simulink model "tanques"  (Simulink 4.00)
settings: Solver=ode45  StartTime=0.0  StopTime=300  MaxStep=0.01  RelTol=1e-3
settings Model: LastModifiedBy=Gui

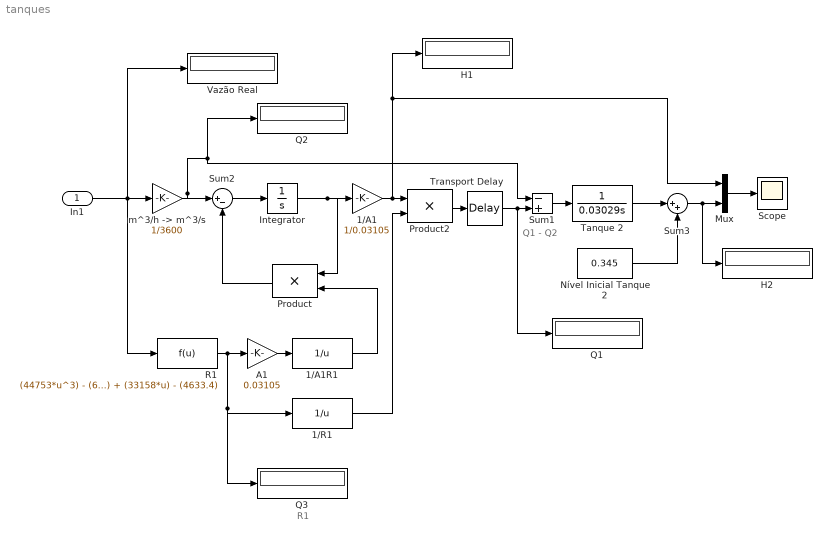
== system tanques ==
  note: Q1 - Q2
  note: R1
  In1 : Inport  Port=1  LatchInput=off
  1/A1 : Gain  Gain=1/0.03105  Multiplication=Element-wise(K.*u)  SaturateOnIntegerOverflow=on
  1/A1R1 : Fcn  Expr=1/u
  1/R1 : Fcn  Expr=1/u
  A1 : Gain  Gain=0.03105  Multiplication=Element-wise(K.*u)  SaturateOnIntegerOverflow=on
  H1 : Display
      settings: Format=short
  H2 : Display
      settings: Format=short
  Integrator : Integrator  ExternalReset=none  InitialConditionSource=internal  InitialCondition=0  LimitOutput=off  UpperSaturationLimit=inf  LowerSaturationLimit=-inf  ShowSaturationPort=off  ShowStatePort=off  AbsoluteTolerance=auto
  Mux : Mux  Inputs=2
  Nível Inicial Tanque 2 : Constant  Value=0.345
  Product : Product  Orientation=left  Inputs=2  Multiplication=Element-wise(.*)  SaturateOnIntegerOverflow=on
  Product2 : Product  Inputs=2  Multiplication=Element-wise(.*)  SaturateOnIntegerOverflow=on
  Q1 : Display
      settings: Format=short
  Q2 : Display
      settings: Format=short
  Q3 : Display
      settings: Format=short
  R1 : Fcn  Expr=(44753*u^3) - (67476*u^2) + (33158*u) - (4633.4)
  Scope : Scope
      settings: TimeRange=auto  YMin=0.161  YMax=0.1715  SaveToWorkspace=off  SaveName=ScopeData  MaxDataPoints=5000
  Sum1 : Sum  Inputs=-+  SaturateOnIntegerOverflow=on
  Sum2 : Sum  Inputs=|+-  SaturateOnIntegerOverflow=on
  Sum3 : Sum  Inputs=|++  SaturateOnIntegerOverflow=on
  Tanque 2 : TransferFcn  Numerator=[1]  Denominator=[0.03029 0]  AbsoluteTolerance=auto  Realization=auto
  Transport Delay : TransportDelay  DelayTime=4.5  InitialInput=0  BufferSize=1024  PadeOrder=0
  Vazão Real : Display
      settings: Format=short
  "m^3/h -> m^3/s" : Gain  Gain=1/3600  Multiplication=Element-wise(K.*u)  SaturateOnIntegerOverflow=on
  wires:
  In1/1 -> "m^3/h -> m^3/s"/1, Vazão Real/1, R1/1
  "m^3/h -> m^3/s"/1 -> Sum2/1, Q2/1, Sum1/1
  Integrator/1 -> Product/1, 1/A1/1
  Product/1 -> Sum2/2
  A1/1 -> 1/A1R1/1
  1/A1R1/1 -> Product/2
  1/A1/1 -> Product2/1, H1/1, Mux/1
  R1/1 -> A1/1, 1/R1/1, Q3/1
  1/R1/1 -> Product2/2
  Sum1/1 -> Tanque 2/1
  Mux/1 -> Scope/1
  Tanque 2/1 -> Sum3/1
  Nível Inicial Tanque 2/1 -> Sum3/2
  Sum3/1 -> Mux/2, H2/1
  Sum2/1 -> Integrator/1
  Product2/1 -> Transport Delay/1
  Transport Delay/1 -> Sum1/2, Q1/1
